simulink model "exercise2_cours"  (R2017a)
settings: Solver=ode15s  StartTime=0.0  StopTime=200000  RelTol=1e-6
undefined symbols (not defined in the file or in its folder): a, delta, Kprime, omega, omegah, omegal
settings Model: Creator=martinguay  LastModifiedBy=martinguay

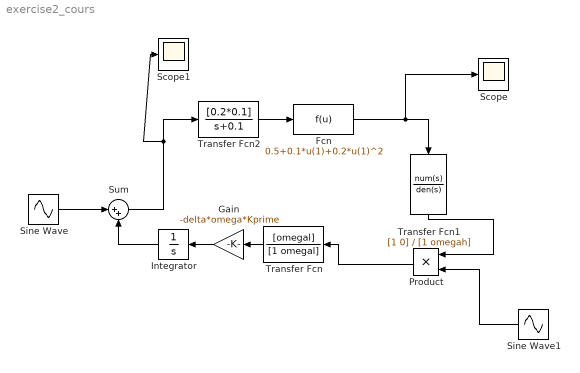
== system exercise2_cours ==
  Fcn : Fcn  Expr=0.5+0.1*u(1)+0.2*u(1)^2
  Gain : Gain  Gain=-delta*omega*Kprime
  Integrator : Integrator
  Product : Product
  Scope : Scope
  Scope1 : Scope
  Sine Wave : Sin  Amplitude=a  Frequency=omega  SampleTime=0
  Sine Wave1 : Sin  Amplitude=1/a  Frequency=omega  SampleTime=0
  Sum : Sum  Inputs=|++
  Transfer Fcn : TransferFcn  Numerator=[omegal]  Denominator=[1 omegal]
  Transfer Fcn1 : TransferFcn  Numerator=[1 0]  Denominator=[1 omegah]
  Transfer Fcn2 : TransferFcn  Numerator=[0.2*0.1]  Denominator=[1 0.1]
  wires:
  Sine Wave/1 -> Sum/1
  Transfer Fcn/1 -> Gain/1
  Sum/1 -> Scope1/1, Transfer Fcn2/1
  Sine Wave1/1 -> Product/2
  Transfer Fcn1/1 -> Product/1
  Product/1 -> Transfer Fcn/1
  Fcn/1 -> Scope/1, Transfer Fcn1/1
  Gain/1 -> Integrator/1
  Integrator/1 -> Sum/2
  Transfer Fcn2/1 -> Fcn/1
